simulink model "MultiSine_Vt"  (R2020a)
settings: Solver=ode45  StartTime=0  StopTime=4.5  FixedStep=0.01  RelTol=0.001  EnableMultiTasking=on
libraries: fmu_me_lib x1
settings Model: Creator=Tin Rabuzin  LastModifiedBy=meagh
settings DataIOCC: LimitDataPoints=on  SaveFormat=Array  ReturnWorkspaceOutputs=off  OutputSaveName=simout  OutputOption=SpecifiedOutputTimes  OutputTimes=[0:0.005:4.5]
settings OptimizationCC: ExpressionDepthLimit=2147483647  LifeSpan=inf
settings DebuggingCC: UnderspecifiedInitializationDetection=Classic  MergeDetectMultiDrivingBlocksExec=none  SolverPrmCheckMsg=warning  StateNameClashWarn=warning  SFUnexpectedBacktrackingDiag=warning  SFNoUnconditionalDefaultTransitionDiag=warning  SFExecutionAtInitializationDiag=none  ArithmeticOperatorsInVariantConditions=warning
settings HardwareCC: ProdBitPerPointer=32  ProdBitPerSizeT=32  ProdBitPerPtrDiffT=32  ProdLargestAtomicFloat=None  ProdIntDivRoundTo=Undefined  ProdEndianess=Unspecified  ProdWordSize=32  ProdHWDeviceType=32-bit Generic
settings ModelReferenceCC: PropagateSignalLabelsOutOfModel=off
settings SFSimCC: SimUseLocalCustomCode=off  CustomCodeUndefinedFunction=UseInterfaceOnly
settings RTWCC: RTWUseLocalCustomCode=off
settings CodeAppCC: StateflowObjectComments=on
settings GRTTargetCC: TargetLangStandard=C89/C90 (ANSI)
settings ConfigComp: CovMetricSettings=dw  CovHtmlReporting=on  CovSaveCumulativeToWorkspaceVar=on  CovSaveSingleToWorkspaceVar=on  CovExternalEMLEnable=off

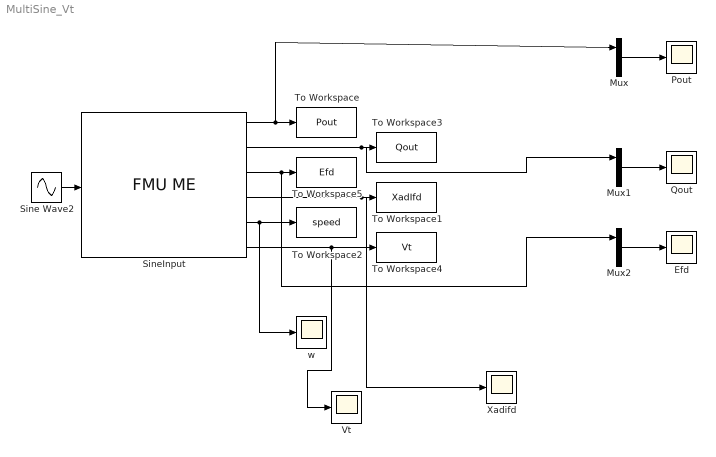
== system MultiSine_Vt ==
  Efd : Scope
  Mux : Mux  Inputs=2
  Mux1 : Mux  Inputs=2
  Mux2 : Mux  Inputs=2
  Pout : Scope
  Qout : Scope
  Sine Wave2 : Sin  Amplitude=0.25  Frequency=1300  SampleTime=0
  SineInput : fmu_me_lib/FMU ME  Description=Simulates an FMU for Model Exchange 1.0 or Model Exchange 2.0.  dummy=0
  To Workspace : ToWorkspace  VariableName=Pout  SaveFormat=Structure With Time  SampleTime=0.005
  To Workspace1 : ToWorkspace  VariableName=XadIfd  SaveFormat=Structure With Time  SampleTime=0.005
  To Workspace2 : ToWorkspace  VariableName=speed  SaveFormat=Structure With Time  SampleTime=0.005
  To Workspace3 : ToWorkspace  VariableName=Qout  SaveFormat=Structure With Time  SampleTime=0.005
  To Workspace4 : ToWorkspace  VariableName=Vt  SaveFormat=Structure With Time  SampleTime=0.005
  To Workspace5 : ToWorkspace  VariableName=Efd  SaveFormat=Structure With Time  SampleTime=0.005
  Vt : Scope
  Xadifd : Scope
  w : Scope
  wires:
  SineInput/1 -> Mux/1, To Workspace/1
  Mux/1 -> Pout/1
  Mux1/1 -> Qout/1
  Mux2/1 -> Efd/1
  SineInput/2 -> Mux1/1, To Workspace3/1
  SineInput/4 -> Xadifd/1, To Workspace1/1
  SineInput/5 -> w/1, To Workspace2/1
  SineInput/6 -> Vt/1, To Workspace4/1
  SineInput/3 -> Mux2/1, To Workspace5/1
  Sine Wave2/1 -> SineInput/1
